simulink model "DCTractionMotorScheme"  (R2022b)
settings: Solver=VariableStepAuto  StartTime=0.0  StopTime=750  RelTol=1e-3
values from neighbouring files (symbols this model uses):
  beta = Ptrac/3/wn^2    (= 0.976675486798)    [DCTractionMotor.m]
  C1 = v_max/wn    (= 0.0530785562633)    [DCTractionMotor.m]
  C2 = wn/vn    (= 5.23333333333)    [DCTractionMotor.m]
  En = eta*Vn    (= 540)    [DCTractionMotor.m]
  Ien = 1    [DCTractionMotor.m]
  J = M*v_max^2/wn^2    (= 73.2506615098)    [DCTractionMotor.m]
  K = Tn/(In*Ien)    (= 1.71974522293)    [DCTractionMotor.m]
  ki_a = wc_i*Ra    (= 42.0576923077)    [DCTractionMotor.m]
  ki_e = wc_e*Re    (= 6000)    [DCTractionMotor.m]
  ki_speed = wc_o*beta    (= 4.88337743399)    [DCTractionMotor.m]
  kp_a = wc_i*La    (= 0.420576923077)    [DCTractionMotor.m]
  kp_e = wc_e*Le    (= 6000)    [DCTractionMotor.m]
  kp_speed = wc_o*J    (= 366.253307549)    [DCTractionMotor.m]
  La = Ra*tau_a    (= 0.000841153846154)    [DCTractionMotor.m]
  Le = Re*tau_e    (= 120)    [DCTractionMotor.m]
  M = Mt+mp*Np    (= 26000)    [DCTractionMotor.m]
  Ra = (Pel-Ptot)/In^2    (= 0.0841153846154)    [DCTractionMotor.m]
  Re = Ven/Ien    (= 120)    [DCTractionMotor.m]
  Tn = Ptot/wn    (= 1226.70441142)    [DCTractionMotor.m]
  Ven = 120    [DCTractionMotor.m]
  Vn = 600    [DCTractionMotor.m]
settings Model: Creator=rubbe  LastModifiedBy=rubbe

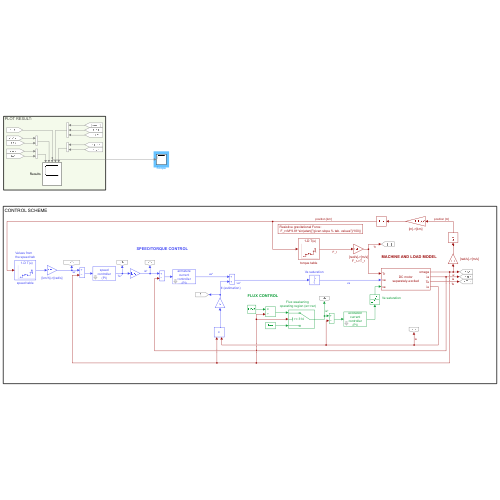
[thumbnail: Simulink's stored preview of the top-level diagram]
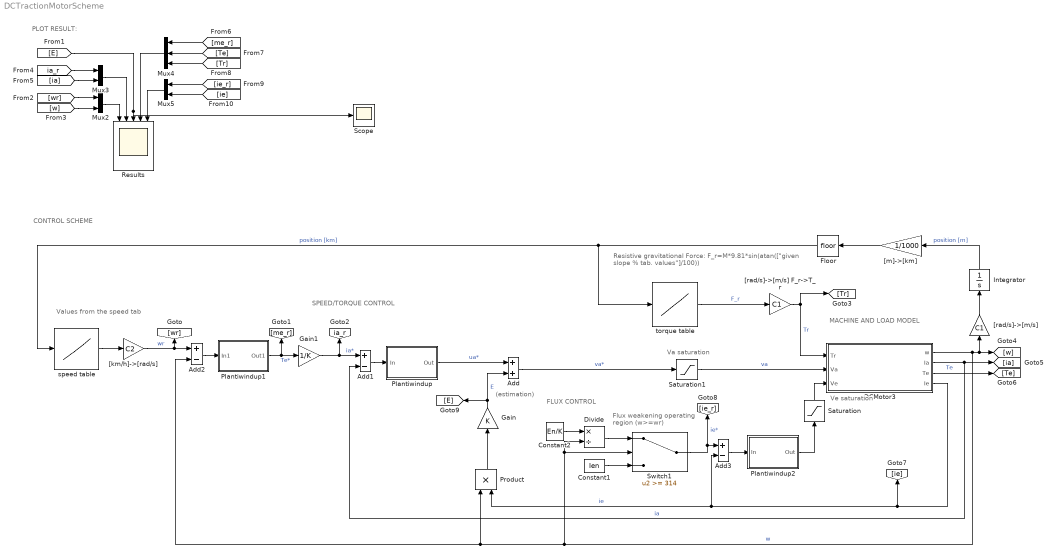
== system DCTractionMotorScheme ==
  note: CONTROL SCHEME
  note: MACHINE AND LOAD MODEL
  note: FLUX CONTROL
  note: SPEED/TORQUE CONTROL
  note: Flux weakening
      | operating region (w>=wr)
  note: (estimation)
  note: PLOT RESULT:
  note: Ve saturation
  note: Values from
      | the speed tab
  note: Va saturation
  note: Resistive gravitational Force:
      |  F_r=M*9.81*sin(atan(["given slope % tab. values"]/100))
  Add : Sum
  Add1 : Sum  Inputs=+-
  Add2 : Sum  Inputs=+-
  Add3 : Sum  Inputs=+-
  Constant1 : Constant  Value=Ien
  Constant2 : Constant  Value=En/K
  DCMotor3 : Subsystem
      mask Display:
      | disp('DC motor\nseparately-excited')
      | port_label('input', 1, 'Tr')
      | port_label('input', 2, 'va')
      | port_label('input', 3, 've')
      | port_label('output', 1, 'omega')
      | port_label('output', 2, 'ia')
      | port_label('output', 3, 'Te')
      | port_label('output', 4, 'ie')
  Divide : Product  Inputs=*/
  Floor : Rounding
  Gain : Gain  Gain=K
  Gain1 : Gain  Gain=1/K
  Integrator : Integrator
  Mux2 : Mux  Inputs=2
  Mux3 : Mux  Inputs=2
  Mux4 : Mux  Inputs=3
  Mux5 : Mux  Inputs=2
  PIantiwindup : Subsystem  mask{Kp=kp_a, Ki=ki_a, sat_up=Vn-En, sat_down=-(Vn-En)}
      mask prompts: sat_up "Upper sat. limit"; sat_down "Lower Sat. Limit"
      mask Display: disp('armature\ncurrent\ncontroller\n(PI)')
  PIantiwindup1 : Subsystem  mask{Kp=kp_speed, Ki=ki_speed, sat_up=Tn, sat_down=-Tn}
      mask prompts: sat_up "Upper sat. limit"; sat_down "Lower Sat. Limit"
      mask Display: disp('speed\ncontroller\n(PI)')
  PIantiwindup2 : Subsystem  mask{Kp=kp_e, Ki=ki_e, sat_up=Ven, sat_down=-Ven}
      mask prompts: sat_up "Upper sat. limit"; sat_down "Lower Sat. Limit"
      mask Display: disp('excitation\ncurrent\ncontroller\n(PI)')
  Product : Product
  Results : Scope  NumInputPorts=5
  Saturation : Saturate  UpperLimit=Ven  LowerLimit=-Ven
  Saturation1 : Saturate  UpperLimit=Vn  LowerLimit=-Vn
  Scope : Scope
  Switch1 : Switch  Threshold=314  SaturateOnIntegerOverflow=off  InputSameDT=off
  "[km/h]->[rad/s]" : Gain  Gain=C2
  "[m]->[km]" : Gain  Gain=1/1000
  "[rad/s]->[m/s]" : Gain  Gain=C1
  "[rad/s]->[m/s] F_r->T_r" : Gain  Gain=C1
  speed table : Lookup_n-D  NumberOfTableDimensions=1  BreakpointsForDimension1=[0 1 3 4 6 8 9 10]  Table=[35 60 60 75 60 60 35 0]  InterpMethod=Flat  InternalRulePriority=Speed  RndMeth=Simplest
  torque table : Lookup_n-D  NumberOfTableDimensions=1  BreakpointsForDimension1=[0 1 3 4 6 8 9 10]  Table=M*9.81*sin(atan([0 0 0.05 0 0 -0.05 0 0]))  InterpMethod=Flat  InternalRulePriority=Speed  RndMeth=Simplest
  tag scope: ia_r=global
  wires:
  torque table/1 -> "[rad/s]->[m/s] F_r->T_r"/1  "F_r"
  Add/1 -> Saturation1/1  "va*"
  [ie] -> Mux5/2
  Saturation1/1 -> DCMotor3/2(Va)  "va"
  "[rad/s]->[m/s] F_r->T_r"/1 -> [Tr], DCMotor3/1(Tr)  "Tr"
  [ia_r] -> Mux3/1
  [ia] -> Mux3/2
  "[m]->[km]"/1 -> Floor/1
  Mux3/1 -> Results/2
  DCMotor3/2(Ia) -> Add1/2, [ia]  "ia"
  Mux2/1 -> Results/1
  Mux4/1 -> Results/4
  [Te] -> Mux4/2
  DCMotor3/1(w) -> [w], "[rad/s]->[m/s]"/1, Divide/2, Switch1/2, Product/1, Add2/2  "w"
  DCMotor3/4(Ie) -> [ie], Add3/2, Product/2  "ie"
  [E] -> Scope/1, Results/3
  Floor/1 -> torque table/1, speed table/1  "position [km]"
  Add3/1 -> PIantiwindup2/1(In)
  DCMotor3/3(Te) -> [Te]  "Te"
  Switch1/1 -> [ie_r], Add3/1  "ie*"
  Saturation/1 -> DCMotor3/3(Ve)
  PIantiwindup2/1(Out) -> Saturation/1
  [w] -> Mux2/2
  Constant1/1 -> Switch1/3
  [ie_r] -> Mux5/1
  Gain/1 -> [E], Add/2  "E"
  Constant2/1 -> Divide/1
  Divide/1 -> Switch1/1
  PIantiwindup1/1(Out1) -> Gain1/1, [me_r]  "Te*"
  [me_r] -> Mux4/1
  "[km/h]->[rad/s]"/1 -> Add2/1, [wr]  "wr"
  "[rad/s]->[m/s]"/1 -> Integrator/1
  [Tr] -> Mux4/3
  Product/1 -> Gain/1
  Gain1/1 -> Add1/1, [ia_r]  "ia*"
  Add2/1 -> PIantiwindup1/1(In1)
  Mux5/1 -> Results/5
  Add1/1 -> PIantiwindup/1(In)
  speed table/1 -> "[km/h]->[rad/s]"/1
  Integrator/1 -> "[m]->[km]"/1  "position [m]"
  PIantiwindup/1(Out) -> Add/1  "ua*"
  [wr] -> Mux2/1

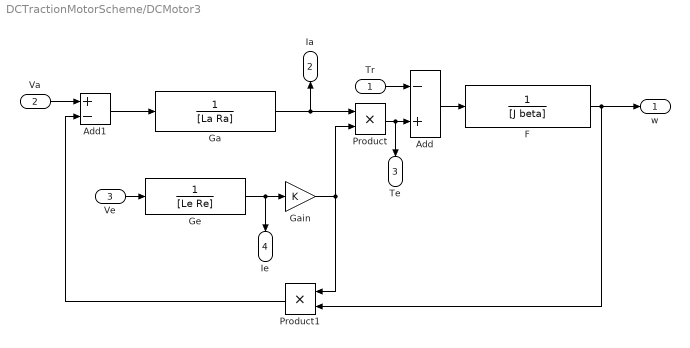
== system DCTractionMotorScheme/DCMotor3 ==
  Tr : Inport
  Va : Inport  Port=2
  Ve : Inport  Port=3
  Add : Sum  Inputs=-+
  Add1 : Sum  Inputs=+-
  F : TransferFcn  Denominator=[J beta]
  Ga : TransferFcn  Denominator=[La Ra]
  Gain : Gain  Gain=K
  Ge : TransferFcn  Denominator=[Le Re]
  Product : Product
  Product1 : Product
  w : Outport  VectorParamsAs1DForOutWhenUnconnected=off
  Ia : Outport  Port=2  VectorParamsAs1DForOutWhenUnconnected=off
  Te : Outport  Port=3  VectorParamsAs1DForOutWhenUnconnected=off
  Ie : Outport  Port=4  VectorParamsAs1DForOutWhenUnconnected=off
  wires:
  Tr/1 -> Add/1
  Add/1 -> F/1
  Gain/1 -> Product1/1, Product/2
  F/1 -> w/1, Product1/2
  Product1/1 -> Add1/2
  Add1/1 -> Ga/1
  Ga/1 -> Ia/1, Product/1
  Product/1 -> Te/1, Add/2
  Ve/1 -> Ge/1
  Va/1 -> Add1/1
  Ge/1 -> Ie/1, Gain/1

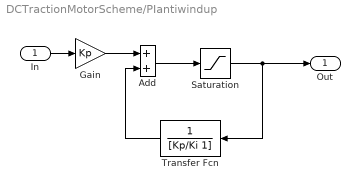
== system DCTractionMotorScheme/PIantiwindup ==
  In : Inport
  Add : Sum
  Gain : Gain  Gain=Kp
  Saturation : Saturate  UpperLimit=sat_up  LowerLimit=sat_down
  Transfer Fcn : TransferFcn  Denominator=[Kp/Ki 1]
  Out : Outport  VectorParamsAs1DForOutWhenUnconnected=off
  wires:
  Saturation/1 -> Out/1, Transfer Fcn/1
  In/1 -> Gain/1
  Gain/1 -> Add/1
  Add/1 -> Saturation/1
  Transfer Fcn/1 -> Add/2

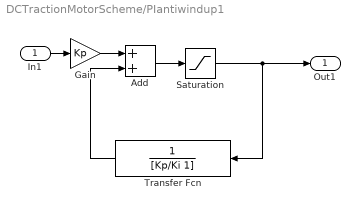
== system DCTractionMotorScheme/PIantiwindup1 ==
  In1 : Inport
  Add : Sum
  Gain : Gain  Gain=Kp
  Saturation : Saturate  UpperLimit=sat_up  LowerLimit=sat_down
  Transfer Fcn : TransferFcn  Denominator=[Kp/Ki 1]
  Out1 : Outport  VectorParamsAs1DForOutWhenUnconnected=off
  wires:
  Transfer Fcn/1 -> Add/2
  Add/1 -> Saturation/1
  Gain/1 -> Add/1
  In1/1 -> Gain/1
  Saturation/1 -> Transfer Fcn/1, Out1/1

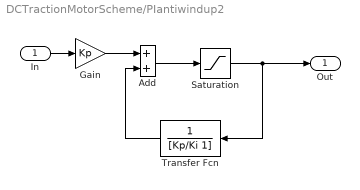
== system DCTractionMotorScheme/PIantiwindup2 ==
  In : Inport
  Add : Sum
  Gain : Gain  Gain=Kp
  Saturation : Saturate  UpperLimit=sat_up  LowerLimit=sat_down
  Transfer Fcn : TransferFcn  Denominator=[Kp/Ki 1]
  Out : Outport  VectorParamsAs1DForOutWhenUnconnected=off
  wires:
  Saturation/1 -> Out/1, Transfer Fcn/1
  In/1 -> Gain/1
  Gain/1 -> Add/1
  Add/1 -> Saturation/1
  Transfer Fcn/1 -> Add/2
